simulink model "sfcndemo_cplx"  (Simulink 7.6)
settings: Solver=FixedStepDiscrete  StartTime=0.0  StopTime=10.0  RelTol=1e-3
Description:
  | Complex Data Handling in I/O and Parameters in a C-MEX S-function
settings Model: Creator=The MathWorks Inc.  ExtModeAutoUpdateStatusClock=off
settings DataIOCC: SaveOutput=off  OutputSaveName=y1,y2,y3,y4
settings OptimizationCC: BlockReduction=off  BooleanDataType=off  InlineInvariantSignals=on  InitFltsAndDblsToZero=on
settings DebuggingCC: SaveWithParameterizedLinksMsg=none  SignalResolutionControl=TryResolveAllWithWarning  SolverPrmCheckMsg=none  MultiTaskDSMMsg=warning  MultiTaskCondExecSysMsg=none
settings HardwareCC: TargetUnknown=on
settings RTWCC: IncludeERTFirstTime=on
settings CodeAppCC: CustomSymbolStrFcn=$F$N$M
settings GRTTargetCC: TargetFcnLib=ansi_tfl_tmw.mat

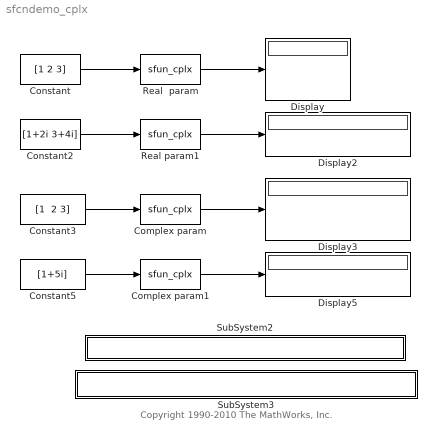
== system sfcndemo_cplx ==
  note: Copyright 1990-2010 The MathWorks, Inc.
  Complex param : S-Function  FunctionName=sfun_cplx  Parameters=[2+3i 4+5i 6+7i]  EnableBusSupport=off
      settings: AttributesFormatString=Param = %<Parameters>
  Complex param1 : S-Function  FunctionName=sfun_cplx  Parameters=[1+3i 7+2i]  EnableBusSupport=off
      settings: AttributesFormatString=Param = %<Parameters>
  Constant : Constant  Value=[1 2 3]  VectorParams1D=off
  Constant2 : Constant  Value=[1+2i 3+4i]  VectorParams1D=off
  Constant3 : Constant  Value="[1  2 3]"  VectorParams1D=off
  Constant5 : Constant  Value=[1+5i]  VectorParams1D=off
  Display{,2..3,5} (4 alike) : Display
  Real  param : S-Function  FunctionName=sfun_cplx  Parameters=5  EnableBusSupport=off
      settings: AttributesFormatString=Param = %<Parameters>
  Real param1 : S-Function  FunctionName=sfun_cplx  Parameters=[5 6]  EnableBusSupport=off
      settings: AttributesFormatString=Param = %<Parameters>
  SubSystem2 : Subsystem  mask{filename=sfun_cplx.c}
      mask init:
      | x=sfundemo_maskdisp;
      settings: AttributesFormatString=\n  OpenFcn=sfundemo_openfcn
      mask Display: disp(x);
  SubSystem3 : Subsystem  mask{filename=sfun_cplx.tlc}
      mask init:
      | x=sfundemo_maskdisp;
      settings: AttributesFormatString=\n  OpenFcn=sfundemo_openfcn
      mask Display: disp(x);
  wires:
  Constant/1 -> Real  param/1
  Real  param/1 -> Display/1
  Constant2/1 -> Real param1/1
  Real param1/1 -> Display2/1
  Constant3/1 -> Complex param/1
  Complex param/1 -> Display3/1
  Constant5/1 -> Complex param1/1
  Complex param1/1 -> Display5/1

== system sfcndemo_cplx/SubSystem2 ==

== system sfcndemo_cplx/SubSystem3 ==
